simulink model "myboost"  (R2016a)
settings: Solver=VariableStepAuto  StartTime=0  StopTime=1  RelTol=1e-3
libraries: powerlib x14, simulink x2, powerlib_meascontrol x1
settings Model: Creator=JookerLoo  LastModifiedBy=JookerLoo

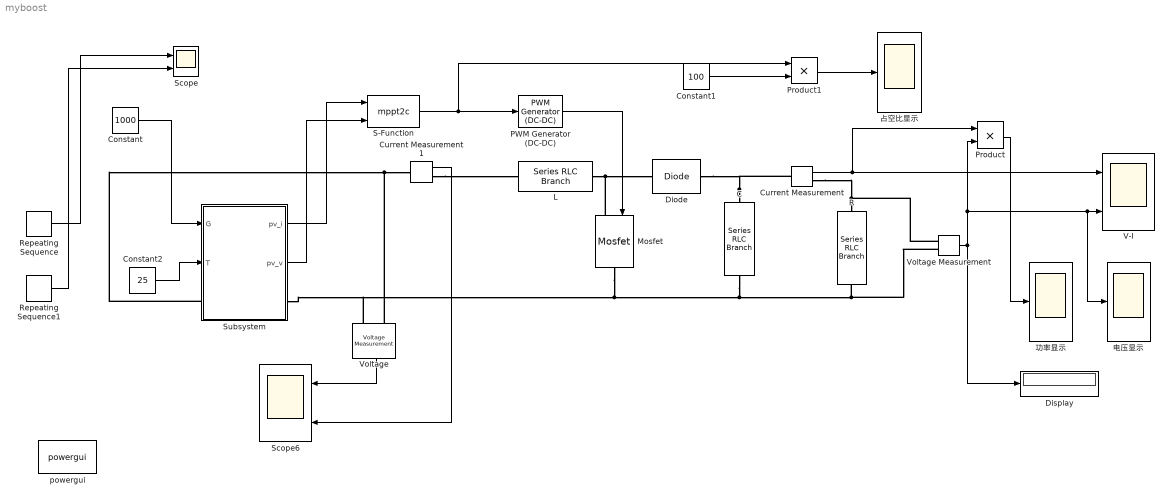
== system myboost ==
  "C " : powerlib/Elements/Series RLC Branch  LConnTagsString=__new0  RConnTagsString=__new0  BranchType=C  Resistance=0  Inductance=1e-3  SetiL0=off  InitialCurrent=0  Capacitance=7.55e-5  Setx0=off  InitialVoltage=0  Measurements=None
  Constant : Constant  Value=1000
  Constant1 : Constant  Value=100
  Constant2 : Constant  Value=25
  Current Measurement : powerlib/Measurements/Current Measurement  PhasorSimulation=off  OutputType=Complex  PSBequivalent=0
  Current Measurement1 : powerlib/Measurements/Current Measurement  PhasorSimulation=off  OutputType=Complex  PSBequivalent=0
  Diode : powerlib/Power Electronics/Diode  Ron=0.001  Lon=0  Vf=0.5  IC=0  UseSnubber=off  Rs=500  Cs=250e-9  Measurements=off
  Display : Display
  L : powerlib/Elements/Series RLC Branch  LConnTagsString=__new0  RConnTagsString=__new0  BranchType=L  Resistance=0  Inductance=8e-5  SetiL0=off  InitialCurrent=0  Capacitance=1e-6  Setx0=off  InitialVoltage=0  Measurements=None
  Mosfet : powerlib/Power Electronics/Mosfet  Ron=0.1  Lon=0  Rd=0.01  Vfd=0.5  IC=0  Rs=1e5  Cs=inf  Measurements=off
  PWM Generator (DC-DC) : powerlib_meascontrol/Pulse & Signal Generators/PWM Generator (DC-DC)  Fsw=50000  Ts=0
  Product : Product
  Product1 : Product
  R : powerlib/Elements/Series RLC Branch  LConnTagsString=__new0  RConnTagsString=__new0  BranchType=R  Resistance=3.6  Inductance=0  SetiL0=off  InitialCurrent=0  Capacitance=0  Setx0=off  InitialVoltage=0  Measurements=None
  Repeating Sequence : simulink/Sources/Repeating Sequence  rep_seq_t=[0 1 2 3 3.5 4 4.5 5]  rep_seq_y=[800 1200 1000 800 900 1000 7000 1000]
  Repeating Sequence1 : simulink/Sources/Repeating Sequence  rep_seq_t=[0 1 2 3 3.5 4 4.5 5]  rep_seq_y=[22 25 22 25 21 28 25 23]
  S-Function : S-Function  FunctionName=mppt2c  SFunctionDeploymentMode=off  EnableBusSupport=off
  Scope : Scope  NumInputPorts=2
  Scope6 : Scope  NumInputPorts=2
  Subsystem : Subsystem
  V-I : Scope  NumInputPorts=2
  "Voltage " : powerlib/Measurements/Voltage Measurement  PhasorSimulation=off  OutputType=Complex  PSBequivalent=0
  Voltage Measurement : powerlib/Measurements/Voltage Measurement  PhasorSimulation=off  OutputType=Complex  PSBequivalent=0
  powergui : powerlib/powergui  Priority=1  SimulationMode=Continuous  SolverType=Tustin/Backward Euler (TBE)  SampleTime=50e-6  frequency=60  SPID=off  DisableSnubberDevices=off  DisableRonSwitches=off  DisableVfSwitches=off  SwTol=0  DisplayEquations=off  Interpol=off  ExternalGateDelay=off  methode=off  Ts=100  FunctionMessages=off  echomessages=off  HookPort=off  EnableUseOfTLC=off  x0status=blocks  frequencyindice=0  Pbase=100e6  ErrMax=1e-4  Iterations=50  UnitsV=kV  UnitsW=MW  buscounter=0  RestoreLinks=warning  ResistiveCurrentMeasurement=off  Frange=[0:2:500]  Ylog=off  Xlog=on  ShowGrid=off  save=off  variable=ZData  structure=0  ZoomFFT=off  StartTime=0.0  cycles=1  DisplayStyle=1  fundamental=60  FreqAxis=off  MaxFrequency=1000  frequencyindicesteady=1  RmsSteady=1  display=off
  功率显示 : Scope
  占空比显示 : Scope
  电压显示 : Scope
  wires:
  Current Measurement/1 -> Product/1, V-I/1
  Subsystem/1(pv_i) -> S-Function/1
  Subsystem/2(pv_v) -> S-Function/2
  PWM Generator (DC-DC)/1 -> Mosfet/1
  S-Function/1 -> Product1/1, PWM Generator (DC-DC)/1
  Current Measurement1/1 -> Scope6/2
  "Voltage "/1 -> Scope6/1
  Voltage Measurement/1 -> Product/2, 电压显示/1, V-I/2, Display/1
  Product/1 -> 功率显示/1
  Constant1/1 -> Product1/2
  Repeating Sequence/1 -> Scope/1
  Product1/1 -> 占空比显示/1
  Constant/1 -> Subsystem/1(G)
  Repeating Sequence1/1 -> Scope/2
  Constant2/1 -> Subsystem/2(T)
  connections:
  L/RConn1 -- Mosfet/LConn1 -- Diode/LConn1
  "C "/LConn1 -- Current Measurement/LConn1 -- Diode/RConn1
  R/RConn1 -- Voltage Measurement/LConn2 -- "Voltage "/LConn2 -- Subsystem/RConn1 -- Mosfet/RConn1 -- "C "/RConn1
  R/LConn1 -- Voltage Measurement/LConn1 -- Current Measurement/RConn1
  "Voltage "/LConn1 -- Subsystem/LConn1 -- Current Measurement1/LConn1
  Current Measurement1/RConn1 -- L/LConn1

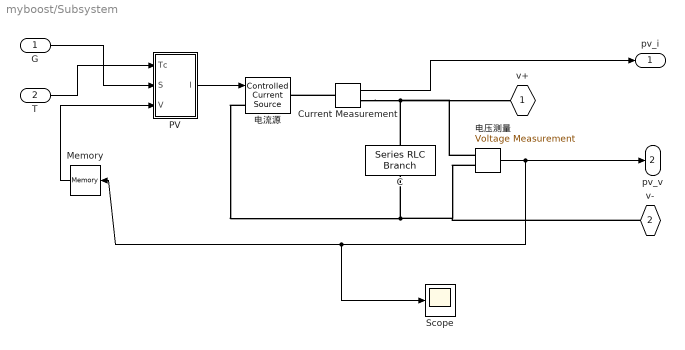
== system myboost/Subsystem ==
  G : Inport
  T : Inport  Port=2
  C : powerlib/Elements/Series RLC Branch  LConnTagsString=__new0  RConnTagsString=__new0  BranchType=C  Resistance=1  Inductance=1e-3  SetiL0=off  InitialCurrent=0  Capacitance=100e-6  Setx0=off  InitialVoltage=0  Measurements=None
  Current Measurement : powerlib/Measurements/Current Measurement  PhasorSimulation=off  OutputType=Complex  PSBequivalent=0
  Memory : Memory
  PV : Subsystem  mask{Im=7.5, Vm=12, Voc=15, Isc=8, Sref=1000, Tref=25, a=0.015, b=0.7, Rs=2}
      mask prompts: Im "最大功率点电流"; Vm "最大功率点电压"; Voc "开路电压"; Isc "短路电流"; Sref "参考光照"; Tref "参考温度"
      mask help: PV_modle
  Scope : Scope
  电压测量 : powerlib/Measurements/Voltage Measurement  PhasorSimulation=off  OutputType=Complex  PSBequivalent=0
  电流源 : powerlib/Electrical Sources/Controlled Current Source  Initialize=on  Source_Type=AC  Amplitude=0  Phase=0  Frequency=0  Measurements=None
  v+ : PMIOPort  Port=1  Side=Left
  v- : PMIOPort  Port=2  Side=Right
  pv_i : Outport
  pv_v : Outport  Port=2
  wires:
  Memory/1 -> PV/3(V)
  PV/1(I) -> 电流源/1
  电压测量/1 -> pv_v/1, Scope/1, Memory/1
  Current Measurement/1 -> pv_i/1
  G/1 -> PV/2(S)
  T/1 -> PV/1(Tc)
  connections:
  Current Measurement/LConn1 -- 电流源/RConn1
  Current Measurement/RConn1 -- 电压测量/LConn1 -- v+/RConn1 -- C/LConn1
  电流源/LConn1 -- 电压测量/LConn2 -- v-/RConn1 -- C/RConn1

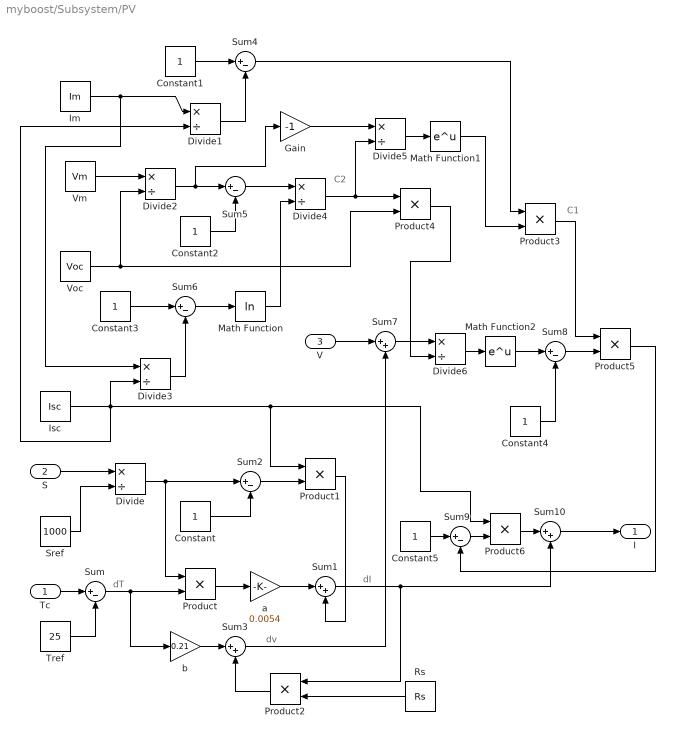
== system myboost/Subsystem/PV ==
  note: C2
  note: dI
  note: dv
  note: dT
  note: C1
  Tc : Inport
  S : Inport  Port=2
  V : Inport  Port=3
  Constant{,1..5} (6 alike) : Constant
  Divide{,1..6} (7 alike) : Product  Inputs=*/
  Gain : Gain  Gain=-1
  Im : Constant  Value=Im
  Isc : Constant  Value=Isc
  Math Function : Math  Operator=log  SaturateOnIntegerOverflow=on
  Math Function1 : Math  SaturateOnIntegerOverflow=on
  Math Function2 : Math  SaturateOnIntegerOverflow=on
  Product{,1..6} (7 alike) : Product  RndMeth=Zero
  Rs : Constant  Value=Rs
  Sref : Constant  Value=1000
  Sum{,2,4..6,8..9} (7 alike) : Sum  Inputs=|+-
  Sum{1,3,7,10} (4 alike) : Sum  Inputs=|++
  Tref : Constant  Value=25
  Vm : Constant  Value=Vm
  Voc : Constant  Value=Voc
  a : Gain  Gain=0.0054
  b : Gain  Gain=0.21
  I : Outport
  wires:
  Tc/1 -> Sum/1
  Tref/1 -> Sum/2
  Sum/1 -> Product/2, b/1
  S/1 -> Divide/1
  Sref/1 -> Divide/2
  Divide/1 -> Product/1, Sum2/1
  Product/1 -> a/1
  Constant/1 -> Sum2/2
  Sum2/1 -> Product1/2
  Product1/1 -> Sum1/2
  a/1 -> Sum1/1
  Sum1/1 -> Product2/1, Sum10/2
  b/1 -> Sum3/1
  Rs/1 -> Product2/2
  Product2/1 -> Sum3/2
  Sum3/1 -> Sum7/2
  Constant1/1 -> Sum4/1
  Im/1 -> Divide3/1, Divide1/1
  Divide1/1 -> Sum4/2
  Vm/1 -> Divide2/1
  Voc/1 -> Divide2/2, Product4/2
  Divide2/1 -> Sum5/1, Gain/1
  Constant2/1 -> Sum5/2
  Constant3/1 -> Sum6/1
  Divide3/1 -> Sum6/2
  Sum6/1 -> Math Function/1
  Sum5/1 -> Divide4/1
  Math Function/1 -> Divide4/2
  Divide4/1 -> Divide5/2, Product4/1
  Gain/1 -> Divide5/1
  Divide5/1 -> Math Function1/1
  Sum4/1 -> Product3/1
  Math Function1/1 -> Product3/2
  Product3/1 -> Product5/1
  Isc/1 -> Product6/1, Product1/1, Divide3/2, Divide1/2
  V/1 -> Sum7/1
  Sum7/1 -> Divide6/1
  Divide6/1 -> Math Function2/1
  Math Function2/1 -> Sum8/1
  Constant4/1 -> Sum8/2
  Sum8/1 -> Product5/2
  Constant5/1 -> Sum9/1
  Product5/1 -> Sum9/2
  Sum9/1 -> Product6/2
  Product6/1 -> Sum10/1
  Product4/1 -> Divide6/2
  Sum10/1 -> I/1
